simulink model "han_ModeChange_DoubleClick"  (R2022b)
settings: Solver=FixedStepAuto  StartTime=0.0  StopTime=inf  FixedStep=0.01  RelTol=1e-3
libraries: simulink x3, spsOnDelayLib x2, dspswit3 x1, arduinolib x1
settings Model: ExtModeTrigDuration=2  Creator=현대오토1  LastModifiedBy=현대오토18
settings OptimizationCC: EnhancedBackFolding=on  PassReuseOutputArgsAs=Individual arguments  ZeroExternalMemoryAtStartup=off  ZeroInternalMemoryAtStartup=off  MaxStackSize=64  OptimizeBlockOrder=speed  DifferentSizesBufferReuse=on  OptimizationCustomize=off  EfficientTunableParamExpr=on
settings DebuggingCC: MultiTaskRateTransMsg=warning  ParameterTunabilityLossMsg=error
settings HardwareCC: ProdBitPerInt=16  ProdBitPerPointer=16  ProdBitPerSizeT=16  ProdBitPerPtrDiffT=16  ProdLargestAtomicFloat=None  ProdWordSize=8  ProdHWDeviceType=Atmel->AVR
settings SFSimCC: MATLABDynamicMemAlloc=off
settings RTWCC: Description=Embedded Coder  SystemTargetFile=ert.tlc  HardwareBoard=Arduino Mega 2560  TLCOptions=-aInlineSetEventsForThisBaseRateFcn=TLC_FALSE -aSuppressMultiTaskScheduler=TLC_FALSE -aRateBasedStepFcn=1  TemplateMakefile=ert_default_tmf  Toolchain=Arduino AVR  BuildConfiguration=Faster Runs
settings CodeAppCC: ForceParamTrailComments=on  IgnoreCustomStorageClasses=off  OperatorAnnotations=on  SimulinkDataObjDesc=on  SFDataObjDesc=on  InsertBlockDesc=on
settings ERTTargetCC: SupportContinuousTime=on  SupportVariableSizeSignals=on  ExtModeTransport=3  ExtModeStaticAlloc=on  ExtModeAutomaticAllocSize=off  ExtModeStaticAllocSize=2048  ExtModeMexFile=ext_xcp  ExtModeIntrfLevel=Level2 - Open

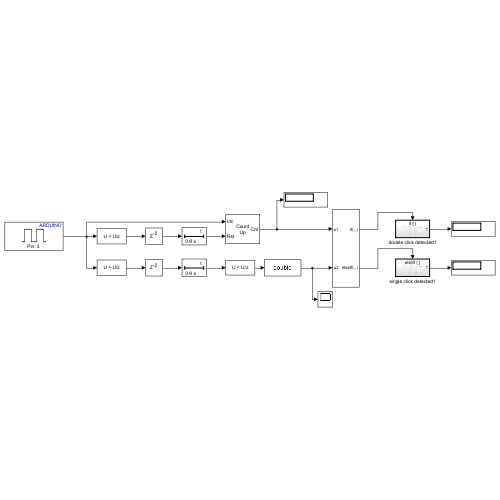
[thumbnail: Simulink's stored preview of the top-level diagram]
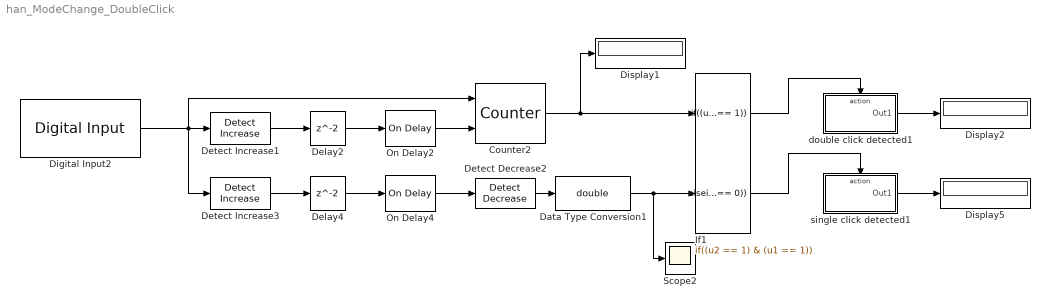
== system han_ModeChange_DoubleClick ==
  Counter2 : dspswit3/Counter  Direction=Up  CountEvent=Rising edge  CounterSize=User defined  MaxCount=255  InitialCount=0  Output=Count  HitValue=32  ResetInput=on  SamplesPerFrame=1  Ts=1  CntDtype=double  HitDtype=Logical
  Data Type Conversion1 : DataTypeConversion  OutDataTypeStr=double  SaturateOnIntegerOverflow=off  RndMeth=Floor
  Delay2 : Delay
  Delay4 : Delay
  Detect Decrease2 : simulink/Logic and Bit Operations/Detect Decrease  vinit=0  OutDataTypeStr=uint8
  Detect Increase1 : simulink/Logic and Bit Operations/Detect Increase  vinit=1  OutDataTypeStr=boolean
  Detect Increase3 : simulink/Logic and Bit Operations/Detect Increase  vinit=1  OutDataTypeStr=boolean
  Digital Input2 : arduinolib/Digital Input  pinNumber=3  mode=Default  Direction=input  SampleTime=0.01  blockPlatform=arduino
  Display1 : Display
  Display2 : Display
  Display5 : Display
  If1 : If  NumInputs=2  IfExpression=(u2 == 1) & (u1 == 1)  ElseIfExpressions=(u2 == 1) & (u1 == 0)  ShowElse=off
  On Delay2 : spsOnDelayLib/On Delay  DelayType=Off delay  delay=0.9  ic=0  Ts=0
  On Delay4 : spsOnDelayLib/On Delay  DelayType=Off delay  delay=0.9  ic=0  Ts=0
  Scope2 : Scope
  double click detected1 : Subsystem  TreatAsAtomicUnit=on
  single click detected1 : Subsystem  TreatAsAtomicUnit=on
  wires:
  Detect Increase1/1 -> Delay2/1
  Delay4/1 -> On Delay4/1
  If1/1 -> double click detected1/Action
  Counter2/1 -> If1/1, Display1/1
  double click detected1/1(Out1) -> Display2/1
  Delay2/1 -> On Delay2/1
  On Delay4/1 -> Detect Decrease2/1
  Detect Decrease2/1 -> Data Type Conversion1/1
  Data Type Conversion1/1 -> If1/2, Scope2/1
  On Delay2/1 -> Counter2/2
  Digital Input2/1 -> Detect Increase1/1, Detect Increase3/1, Counter2/1
  Detect Increase3/1 -> Delay4/1
  If1/2 -> single click detected1/Action
  single click detected1/1(Out1) -> Display5/1

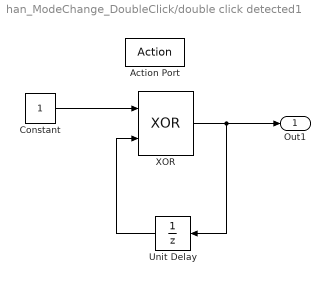
== system han_ModeChange_DoubleClick/double click detected1 ==
  Action Port : ActionPort  ActionPortLabel=if((u2 == 1) & (u1 == 1))
  Constant : Constant
  Unit Delay : UnitDelay  SampleTime=-1  HasFrameUpgradeWarning=on
  XOR : Logic  Operator=XOR  IconShape=distinctive  AllPortsSameDT=off  OutDataTypeStr=boolean
  Out1 : Outport
  wires:
  Unit Delay/1 -> XOR/2
  XOR/1 -> Out1/1, Unit Delay/1
  Constant/1 -> XOR/1

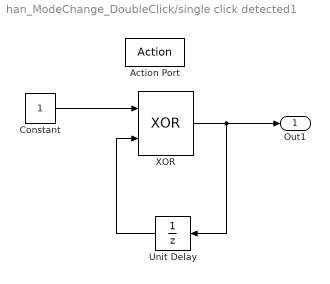
== system han_ModeChange_DoubleClick/single click detected1 ==
  Action Port : ActionPort  ActionPortLabel=elseif((u2 == 1) & (u1 == 0))
  Constant : Constant
  Unit Delay : UnitDelay  SampleTime=-1  HasFrameUpgradeWarning=on
  XOR : Logic  Operator=XOR  IconShape=distinctive  AllPortsSameDT=off  OutDataTypeStr=boolean
  Out1 : Outport
  wires:
  Constant/1 -> XOR/1
  XOR/1 -> Unit Delay/1, Out1/1
  Unit Delay/1 -> XOR/2
